simulink model "Feeder_1"  (Simulink 8.8)
settings: Solver=ode4  StartTime=0.0  StopTime=inf  FixedStep=Ts  RelTol=1e-3  EnableMultiTasking=on
PreLoadFcn:
  | Ts=125e-6;Core_Num = 0; np=1; nq=1; Vmin=.9;
PostLoadFcn:
  | Ts=125e-6;Core_Num = 0; np=1; nq=1; Vmin=.9;
InitFcn:
  | Ts=125e-6;Core_Num = 0; np=1; nq=1; Vmin=.9;
undefined symbols (not defined in the file or in its folder): another_event_name, DiscIntNeverNeededParam, I, j, Left, my_event_name, Right, type, V, X
libraries: powerlib x316, powerlib_meascontrol x227, simulink_extras x78, simulink x25, rtio_generic_c37_118 x22, ssn_lib x9, rtlab x6, powerlib_extras x3, artemis x1, rtio_opalrt_ml605ex1 x1, rtio_spectracom x1, rtio_generic_ethernet x1
(part 10 of 14)

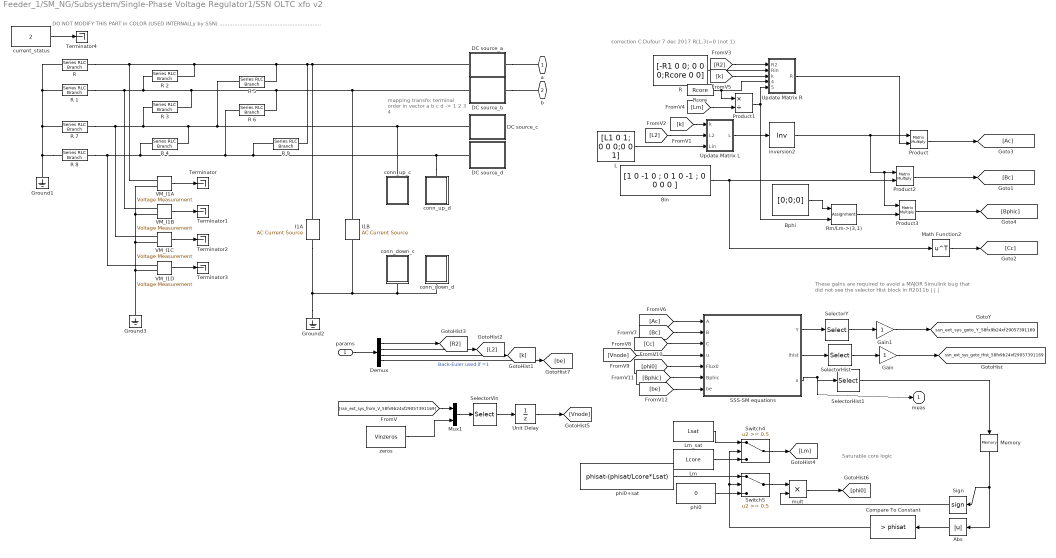
== system Feeder_1/SM_NG/Subsystem/Single-Phase Voltage Regulator1/SSN OLTC xfo v2 ==
  note: correction C.Dufour 7 dec 2017 R(1,3)=0 (not 1)
  note: These gains are required to avoid a MAJOR Simulink bug
      | that did not see the selector Hist block in R2011b
      | |
      | |
      | |
  note: Saturable core logic
  note: DO NOT MODIFY THIS PART in COLOR (USED INTERNALLy by SSN) .............................................................
  note: mapping transfo:
      | terminal    order in vector
      | a b c d -> 1 2 3 4
  params : Inport
  Abs : Abs
  Bin : Constant  Value="[1 0 -1  0 ; 0 1 0 -1 ; 0 0 0 0 ]"
  Bphi : Constant  Value=[0;0;0]  VectorParams1D=off
  Compare To Constant : simulink/Logic and Bit Operations/Compare To Constant  relop=>  const=phisat  OutDataTypeStr=uint8
  DC source_a : Subsystem  mask(SSN nodal point interface: DC-source){}
  DC source_b : Subsystem  mask(SSN nodal point interface: DC-source){}
  DC source_c : Subsystem  mask(SSN nodal point interface: DC-source){}
  DC source_d : Subsystem  mask(SSN nodal point interface: DC-source){}
  Demux : Demux
  Gain : Gain
  Gain1 : Gain
  Ground1 : powerlib/Elements/Ground  LConnTagsString=a
  Ground2 : powerlib/Elements/Ground  LConnTagsString=a
  Ground3 : powerlib/Elements/Ground  LConnTagsString=a
  I1A : powerlib/Electrical Sources/AC Current Source  Amplitude=0  Phase=0  Frequency=1928.3746  SampleTime=0  Measurements=None
  I1B : powerlib/Electrical Sources/AC Current Source  Amplitude=0  Phase=0  Frequency=1928.3746  SampleTime=0  Measurements=None
  L : Constant  Value=[L1 0 1; 0 0 0;0 0 1]
  Lm : Constant  Value=Lcore
  Lm_sat : Constant  Value=Lsat
  Math Function2 : Math  Operator=transpose  SaturateOnIntegerOverflow=on
  Memory : Memory
  Mux1 : Mux  Inputs=2
  Product : Product  Multiplication=Matrix(*)  RndMeth=Zero
  Product1 : Product  Inputs=*/  RndMeth=Zero
  Product2 : Product  Multiplication=Matrix(*)  RndMeth=Zero
  Product3 : Product  Multiplication=Matrix(*)  RndMeth=Zero
  R : Constant  Value=[-R1 0 0; 0 0 0;Rcore 0 0]
  R {,1..9} (10 alike) : powerlib/Elements/Series RLC Branch  LConnTagsString=__new0  RConnTagsString=__new0  BranchType=R  Resistance=1.23456789  Inductance=.5  SetiL0=off  InitialCurrent=0  Capacitance=1.0  Setx0=off  InitialVoltage=0  Measurements=None
  Rcore : Constant  Value=Rcore
  "Rm/Lm->(3,1) " : Assignment  NumberOfDimensions=2  IndexOptions=Index vector (dialog),Index vector (dialog)  Indices=3,1  OutputSizes=1,1
  SSS-SM equations : Subsystem
  SelectorHist : Selector  InputPortWidth=4  IndexOptions=Index vector (dialog)  Indices=hist_sel  OutputSizes=1
  SelectorHist1 : Selector  InputPortWidth=3  IndexOptions=Index vector (dialog)  Indices=3  OutputSizes=1
  SelectorVin : Selector  InputPortWidth=5  IndexOptions=Index vector (dialog)  Indices=vin_sel  OutputSizes=1
  SelectorY : Selector  NumberOfDimensions=2  InputPortWidth=4  IndexOptions=Index vector (dialog),Index vector (dialog)  Indices=hist_sel,hist_sel  OutputSizes=1,1
  Sign : Signum
  Switch4 : Switch  Threshold=0.5
  Switch5 : Switch  Threshold=0.5
  Terminator{,1..4} (5 alike) : Terminator
  Unit Delay : UnitDelay  SampleTime=Ts
  Update Matrix L : Subsystem
  Update Matrix R : Subsystem
  VM_I1A : powerlib/Measurements/Voltage Measurement  PhasorSimulation=off  OutputType=Complex  PSBequivalent=0
  VM_I1B : powerlib/Measurements/Voltage Measurement  PhasorSimulation=off  OutputType=Complex  PSBequivalent=0
  VM_I1C : powerlib/Measurements/Voltage Measurement  PhasorSimulation=off  OutputType=Complex  PSBequivalent=0
  VM_I1D : powerlib/Measurements/Voltage Measurement  PhasorSimulation=off  OutputType=Complex  PSBequivalent=0
  conn_down_c : Subsystem
  conn_down_d : Subsystem
  conn_up_c : Subsystem
  conn_up_d : Subsystem
  current_status : Constant  Value=2
  inversion2 : Product  Inputs=/  Multiplication=Matrix(*)  RndMeth=Zero
  mult : Product
  phi0 : Constant  Value=0
  phi0+sat : Constant  Value=phisat-(phisat/Lcore*Lsat)
  zeros : Constant  Value=Vinzeros
  a : PMIOPort  Port=1  Side=Left
  b : PMIOPort  Port=2  Side=Right
  meas : Outport  InitialOutput=0
  tag scope: ssn_ext_sys_goto_Hist_58fx9b24xf29057391169=global, ssn_ext_sys_goto_Y_58fx9b24xf29057391169=global
  wires:
  Gain1/1 -> [ssn_ext_sys_goto_Y_58fx9b24xf29057391169]
  Gain/1 -> [ssn_ext_sys_goto_Hist_58fx9b24xf29057391169]
  Sign/1 -> mult/2
  mult/1 -> [phi0]
  Switch5/1 -> mult/1
  Unit Delay/1 -> [Vnode]
  params/1 -> Demux/1
  Demux/1 -> [R2]
  Demux/2 -> [L2]
  Demux/3 -> [k]
  Abs/1 -> Compare To Constant/1
  Lm_sat/1 -> Switch4/1
  Lm/1 -> Switch4/3
  Memory/1 -> Abs/1, Sign/1
  phi0/1 -> Switch5/3
  phi0+sat/1 -> Switch5/1
  Switch4/1 -> [Lm]
  Compare To Constant/1 -> Switch4/2, Switch5/2
  [ssn_ext_sys_from_V_58fx9b24xf29057391169] -> Mux1/1
  zeros/1 -> Mux1/2
  SelectorVin/1 -> Unit Delay/1
  Mux1/1 -> SelectorVin/1
  current_status/1 -> Terminator4/1
  VM_I1D/1 -> Terminator3/1
  VM_I1C/1 -> Terminator2/1
  VM_I1B/1 -> Terminator1/1
  VM_I1A/1 -> Terminator/1
  L/1 -> Update Matrix L/3(Lin)
  [k] -> Update Matrix L/1(k)
  [L2] -> Update Matrix L/2(L2)
  Update Matrix L/1(L) -> inversion2/1
  R/1 -> Update Matrix R/2(Rin)
  [R2] -> Update Matrix R/1(R2)
  [k] -> Update Matrix R/3(k)
  Rcore/1 -> Update Matrix R/4(Rcore), Product1/1
  inversion2/1 -> Product2/1, Product3/1, Product/1
  [Lm] -> Product1/2
  Product1/1 -> Update Matrix R/5(Rcore/Lcore), "Rm/Lm->(3,1) "/2
  Bin/1 -> Math Function2/1, Product2/2
  Math Function2/1 -> [Cc]
  [Ac] -> SSS-SM equations/1(A)
  [Bc] -> SSS-SM equations/2(B)
  [Cc] -> SSS-SM equations/3(C)
  [Vnode] -> SSS-SM equations/4(u)
  [phi0] -> SSS-SM equations/5(Flux0)
  Bphi/1 -> "Rm/Lm->(3,1) "/1
  [Bphic] -> SSS-SM equations/6(Bphic)
  Product2/1 -> [Bc]
  "Rm/Lm->(3,1) "/1 -> Product3/2
  Update Matrix R/1(R) -> Product/2
  Product/1 -> [Ac]
  Product3/1 -> [Bphic]
  SSS-SM equations/3(x) -> SelectorHist1/1, meas/1
  SelectorHist1/1 -> Memory/1
  [be] -> SSS-SM equations/7(be)
  Demux/4 -> [be]  "Back-Euler used if =1"
  SSS-SM equations/2(Ihist) -> SelectorHist/1
  SSS-SM equations/1(Y) -> SelectorY/1
  SelectorY/1 -> Gain1/1
  SelectorHist/1 -> Gain/1
  connections:
  R 5/RConn1 -- VM_I1A/LConn1 -- "R "/RConn1 -- R 2/RConn1 -- I1A/RConn1 -- DC source_a/LConn1 -- R 9/RConn1
  R 3/RConn1 -- VM_I1B/LConn1 -- R 1/RConn1 -- R 2/LConn1 -- I1B/RConn1 -- DC source_b/LConn1 -- R 6/RConn1
  R 4/RConn1 -- VM_I1C/LConn1 -- R 7/RConn1 -- R 3/LConn1 -- conn_up_c/LConn1 -- DC source_c/LConn1 -- R 5/LConn1
  conn_up_d/LConn1 -- DC source_d/LConn1 -- R 9/LConn1 -- R 6/LConn1 -- VM_I1D/LConn1 -- R 8/RConn1 -- R 4/LConn1
  Ground3/LConn1 -- VM_I1C/LConn2 -- VM_I1A/LConn2 -- VM_I1B/LConn2 -- VM_I1D/LConn2
  DC source_b/RConn1 -- b/RConn1
  Ground2/LConn1 -- I1A/LConn1 -- I1B/LConn1 -- conn_down_c/RConn1 -- conn_down_d/RConn1
  DC source_a/RConn1 -- a/RConn1
  R 8/LConn1 -- Ground1/LConn1 -- R 7/LConn1 -- R 1/LConn1 -- "R "/LConn1

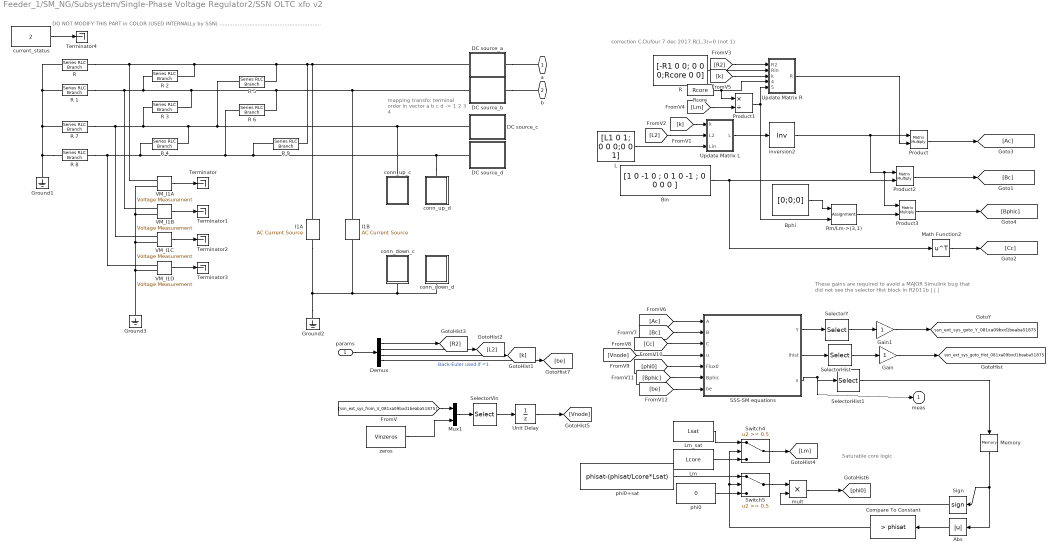
== system Feeder_1/SM_NG/Subsystem/Single-Phase Voltage Regulator2/SSN OLTC xfo v2 ==
  note: correction C.Dufour 7 dec 2017 R(1,3)=0 (not 1)
  note: These gains are required to avoid a MAJOR Simulink bug
      | that did not see the selector Hist block in R2011b
      | |
      | |
      | |
  note: Saturable core logic
  note: DO NOT MODIFY THIS PART in COLOR (USED INTERNALLy by SSN) .............................................................
  note: mapping transfo:
      | terminal    order in vector
      | a b c d -> 1 2 3 4
  params : Inport
  Abs : Abs
  Bin : Constant  Value="[1 0 -1  0 ; 0 1 0 -1 ; 0 0 0 0 ]"
  Bphi : Constant  Value=[0;0;0]  VectorParams1D=off
  Compare To Constant : simulink/Logic and Bit Operations/Compare To Constant  relop=>  const=phisat  OutDataTypeStr=uint8
  DC source_a : Subsystem  mask(SSN nodal point interface: DC-source){}
  DC source_b : Subsystem  mask(SSN nodal point interface: DC-source){}
  DC source_c : Subsystem  mask(SSN nodal point interface: DC-source){}
  DC source_d : Subsystem  mask(SSN nodal point interface: DC-source){}
  Demux : Demux
  Gain : Gain
  Gain1 : Gain
  Ground1 : powerlib/Elements/Ground  LConnTagsString=a
  Ground2 : powerlib/Elements/Ground  LConnTagsString=a
  Ground3 : powerlib/Elements/Ground  LConnTagsString=a
  I1A : powerlib/Electrical Sources/AC Current Source  Amplitude=0  Phase=0  Frequency=1928.3746  SampleTime=0  Measurements=None
  I1B : powerlib/Electrical Sources/AC Current Source  Amplitude=0  Phase=0  Frequency=1928.3746  SampleTime=0  Measurements=None
  L : Constant  Value=[L1 0 1; 0 0 0;0 0 1]
  Lm : Constant  Value=Lcore
  Lm_sat : Constant  Value=Lsat
  Math Function2 : Math  Operator=transpose  SaturateOnIntegerOverflow=on
  Memory : Memory
  Mux1 : Mux  Inputs=2
  Product : Product  Multiplication=Matrix(*)  RndMeth=Zero
  Product1 : Product  Inputs=*/  RndMeth=Zero
  Product2 : Product  Multiplication=Matrix(*)  RndMeth=Zero
  Product3 : Product  Multiplication=Matrix(*)  RndMeth=Zero
  R : Constant  Value=[-R1 0 0; 0 0 0;Rcore 0 0]
  R {,1..9} (10 alike) : powerlib/Elements/Series RLC Branch  LConnTagsString=__new0  RConnTagsString=__new0  BranchType=R  Resistance=1.23456789  Inductance=.5  SetiL0=off  InitialCurrent=0  Capacitance=1.0  Setx0=off  InitialVoltage=0  Measurements=None
  Rcore : Constant  Value=Rcore
  "Rm/Lm->(3,1) " : Assignment  NumberOfDimensions=2  IndexOptions=Index vector (dialog),Index vector (dialog)  Indices=3,1  OutputSizes=1,1
  SSS-SM equations : Subsystem
  SelectorHist : Selector  InputPortWidth=4  IndexOptions=Index vector (dialog)  Indices=hist_sel  OutputSizes=1
  SelectorHist1 : Selector  InputPortWidth=3  IndexOptions=Index vector (dialog)  Indices=3  OutputSizes=1
  SelectorVin : Selector  InputPortWidth=5  IndexOptions=Index vector (dialog)  Indices=vin_sel  OutputSizes=1
  SelectorY : Selector  NumberOfDimensions=2  InputPortWidth=4  IndexOptions=Index vector (dialog),Index vector (dialog)  Indices=hist_sel,hist_sel  OutputSizes=1,1
  Sign : Signum
  Switch4 : Switch  Threshold=0.5
  Switch5 : Switch  Threshold=0.5
  Terminator{,1..4} (5 alike) : Terminator
  Unit Delay : UnitDelay  SampleTime=Ts
  Update Matrix L : Subsystem
  Update Matrix R : Subsystem
  VM_I1A : powerlib/Measurements/Voltage Measurement  PhasorSimulation=off  OutputType=Complex  PSBequivalent=0
  VM_I1B : powerlib/Measurements/Voltage Measurement  PhasorSimulation=off  OutputType=Complex  PSBequivalent=0
  VM_I1C : powerlib/Measurements/Voltage Measurement  PhasorSimulation=off  OutputType=Complex  PSBequivalent=0
  VM_I1D : powerlib/Measurements/Voltage Measurement  PhasorSimulation=off  OutputType=Complex  PSBequivalent=0
  conn_down_c : Subsystem
  conn_down_d : Subsystem
  conn_up_c : Subsystem
  conn_up_d : Subsystem
  current_status : Constant  Value=2
  inversion2 : Product  Inputs=/  Multiplication=Matrix(*)  RndMeth=Zero
  mult : Product
  phi0 : Constant  Value=0
  phi0+sat : Constant  Value=phisat-(phisat/Lcore*Lsat)
  zeros : Constant  Value=Vinzeros
  a : PMIOPort  Port=1  Side=Left
  b : PMIOPort  Port=2  Side=Right
  meas : Outport  InitialOutput=0
  tag scope: ssn_ext_sys_goto_Hist_081xa09bxd1beaba51875=global, ssn_ext_sys_goto_Y_081xa09bxd1beaba51875=global
  wires:
  Gain1/1 -> [ssn_ext_sys_goto_Y_081xa09bxd1beaba51875]
  Gain/1 -> [ssn_ext_sys_goto_Hist_081xa09bxd1beaba51875]
  Sign/1 -> mult/2
  mult/1 -> [phi0]
  Switch5/1 -> mult/1
  Unit Delay/1 -> [Vnode]
  params/1 -> Demux/1
  Demux/1 -> [R2]
  Demux/2 -> [L2]
  Demux/3 -> [k]
  Abs/1 -> Compare To Constant/1
  Lm_sat/1 -> Switch4/1
  Lm/1 -> Switch4/3
  Memory/1 -> Abs/1, Sign/1
  phi0/1 -> Switch5/3
  phi0+sat/1 -> Switch5/1
  Switch4/1 -> [Lm]
  Compare To Constant/1 -> Switch4/2, Switch5/2
  [ssn_ext_sys_from_V_081xa09bxd1beaba51875] -> Mux1/1
  zeros/1 -> Mux1/2
  SelectorVin/1 -> Unit Delay/1
  Mux1/1 -> SelectorVin/1
  current_status/1 -> Terminator4/1
  VM_I1D/1 -> Terminator3/1
  VM_I1C/1 -> Terminator2/1
  VM_I1B/1 -> Terminator1/1
  VM_I1A/1 -> Terminator/1
  L/1 -> Update Matrix L/3(Lin)
  [k] -> Update Matrix L/1(k)
  [L2] -> Update Matrix L/2(L2)
  Update Matrix L/1(L) -> inversion2/1
  R/1 -> Update Matrix R/2(Rin)
  [R2] -> Update Matrix R/1(R2)
  [k] -> Update Matrix R/3(k)
  Rcore/1 -> Update Matrix R/4(Rcore), Product1/1
  inversion2/1 -> Product2/1, Product3/1, Product/1
  [Lm] -> Product1/2
  Product1/1 -> Update Matrix R/5(Rcore/Lcore), "Rm/Lm->(3,1) "/2
  Bin/1 -> Math Function2/1, Product2/2
  Math Function2/1 -> [Cc]
  [Ac] -> SSS-SM equations/1(A)
  [Bc] -> SSS-SM equations/2(B)
  [Cc] -> SSS-SM equations/3(C)
  [Vnode] -> SSS-SM equations/4(u)
  [phi0] -> SSS-SM equations/5(Flux0)
  Bphi/1 -> "Rm/Lm->(3,1) "/1
  [Bphic] -> SSS-SM equations/6(Bphic)
  Product2/1 -> [Bc]
  "Rm/Lm->(3,1) "/1 -> Product3/2
  Update Matrix R/1(R) -> Product/2
  Product/1 -> [Ac]
  Product3/1 -> [Bphic]
  SSS-SM equations/3(x) -> SelectorHist1/1, meas/1
  SelectorHist1/1 -> Memory/1
  [be] -> SSS-SM equations/7(be)
  Demux/4 -> [be]  "Back-Euler used if =1"
  SSS-SM equations/2(Ihist) -> SelectorHist/1
  SSS-SM equations/1(Y) -> SelectorY/1
  SelectorY/1 -> Gain1/1
  SelectorHist/1 -> Gain/1
  connections:
  R 5/RConn1 -- VM_I1A/LConn1 -- "R "/RConn1 -- R 2/RConn1 -- I1A/RConn1 -- DC source_a/LConn1 -- R 9/RConn1
  R 3/RConn1 -- VM_I1B/LConn1 -- R 1/RConn1 -- R 2/LConn1 -- I1B/RConn1 -- DC source_b/LConn1 -- R 6/RConn1
  R 4/RConn1 -- VM_I1C/LConn1 -- R 7/RConn1 -- R 3/LConn1 -- conn_up_c/LConn1 -- DC source_c/LConn1 -- R 5/LConn1
  conn_up_d/LConn1 -- DC source_d/LConn1 -- R 9/LConn1 -- R 6/LConn1 -- VM_I1D/LConn1 -- R 8/RConn1 -- R 4/LConn1
  Ground3/LConn1 -- VM_I1C/LConn2 -- VM_I1A/LConn2 -- VM_I1B/LConn2 -- VM_I1D/LConn2
  DC source_b/RConn1 -- b/RConn1
  Ground2/LConn1 -- I1A/LConn1 -- I1B/LConn1 -- conn_down_c/RConn1 -- conn_down_d/RConn1
  DC source_a/RConn1 -- a/RConn1
  R 8/LConn1 -- Ground1/LConn1 -- R 7/LConn1 -- R 1/LConn1 -- "R "/LConn1

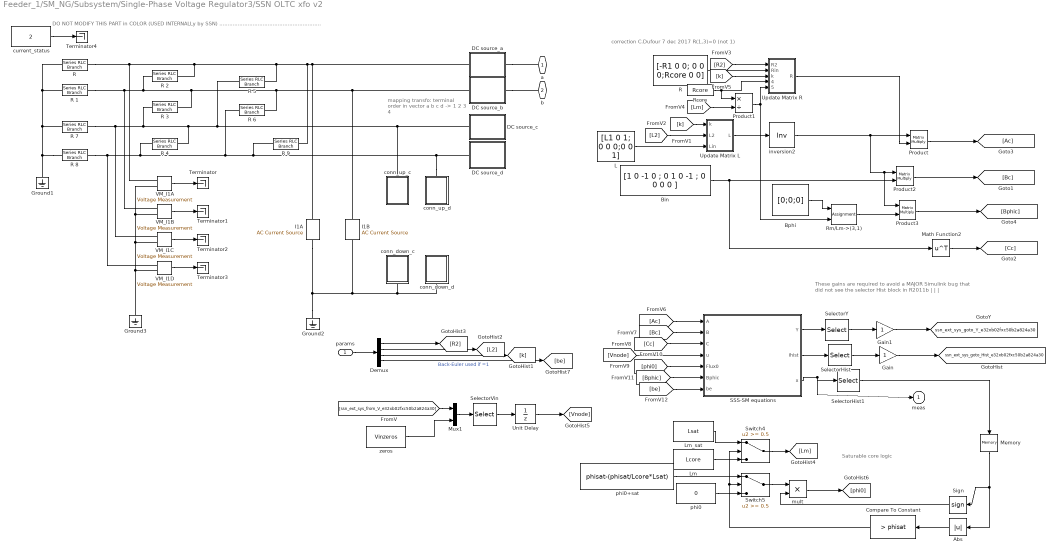
== system Feeder_1/SM_NG/Subsystem/Single-Phase Voltage Regulator3/SSN OLTC xfo v2 ==
  note: correction C.Dufour 7 dec 2017 R(1,3)=0 (not 1)
  note: These gains are required to avoid a MAJOR Simulink bug
      | that did not see the selector Hist block in R2011b
      | |
      | |
      | |
  note: Saturable core logic
  note: DO NOT MODIFY THIS PART in COLOR (USED INTERNALLy by SSN) .............................................................
  note: mapping transfo:
      | terminal    order in vector
      | a b c d -> 1 2 3 4
  params : Inport
  Abs : Abs
  Bin : Constant  Value="[1 0 -1  0 ; 0 1 0 -1 ; 0 0 0 0 ]"
  Bphi : Constant  Value=[0;0;0]  VectorParams1D=off
  Compare To Constant : simulink/Logic and Bit Operations/Compare To Constant  relop=>  const=phisat  OutDataTypeStr=uint8
  DC source_a : Subsystem  mask(SSN nodal point interface: DC-source){}
  DC source_b : Subsystem  mask(SSN nodal point interface: DC-source){}
  DC source_c : Subsystem  mask(SSN nodal point interface: DC-source){}
  DC source_d : Subsystem  mask(SSN nodal point interface: DC-source){}
  Demux : Demux
  Gain : Gain
  Gain1 : Gain
  Ground1 : powerlib/Elements/Ground  LConnTagsString=a
  Ground2 : powerlib/Elements/Ground  LConnTagsString=a
  Ground3 : powerlib/Elements/Ground  LConnTagsString=a
  I1A : powerlib/Electrical Sources/AC Current Source  Amplitude=0  Phase=0  Frequency=1928.3746  SampleTime=0  Measurements=None
  I1B : powerlib/Electrical Sources/AC Current Source  Amplitude=0  Phase=0  Frequency=1928.3746  SampleTime=0  Measurements=None
  L : Constant  Value=[L1 0 1; 0 0 0;0 0 1]
  Lm : Constant  Value=Lcore
  Lm_sat : Constant  Value=Lsat
  Math Function2 : Math  Operator=transpose  SaturateOnIntegerOverflow=on
  Memory : Memory
  Mux1 : Mux  Inputs=2
  Product : Product  Multiplication=Matrix(*)  RndMeth=Zero
  Product1 : Product  Inputs=*/  RndMeth=Zero
  Product2 : Product  Multiplication=Matrix(*)  RndMeth=Zero
  Product3 : Product  Multiplication=Matrix(*)  RndMeth=Zero
  R : Constant  Value=[-R1 0 0; 0 0 0;Rcore 0 0]
  R {,1..9} (10 alike) : powerlib/Elements/Series RLC Branch  LConnTagsString=__new0  RConnTagsString=__new0  BranchType=R  Resistance=1.23456789  Inductance=.5  SetiL0=off  InitialCurrent=0  Capacitance=1.0  Setx0=off  InitialVoltage=0  Measurements=None
  Rcore : Constant  Value=Rcore
  "Rm/Lm->(3,1) " : Assignment  NumberOfDimensions=2  IndexOptions=Index vector (dialog),Index vector (dialog)  Indices=3,1  OutputSizes=1,1
  SSS-SM equations : Subsystem
  SelectorHist : Selector  InputPortWidth=4  IndexOptions=Index vector (dialog)  Indices=hist_sel  OutputSizes=1
  SelectorHist1 : Selector  InputPortWidth=3  IndexOptions=Index vector (dialog)  Indices=3  OutputSizes=1
  SelectorVin : Selector  InputPortWidth=5  IndexOptions=Index vector (dialog)  Indices=vin_sel  OutputSizes=1
  SelectorY : Selector  NumberOfDimensions=2  InputPortWidth=4  IndexOptions=Index vector (dialog),Index vector (dialog)  Indices=hist_sel,hist_sel  OutputSizes=1,1
  Sign : Signum
  Switch4 : Switch  Threshold=0.5
  Switch5 : Switch  Threshold=0.5
  Terminator{,1..4} (5 alike) : Terminator
  Unit Delay : UnitDelay  SampleTime=Ts
  Update Matrix L : Subsystem
  Update Matrix R : Subsystem
  VM_I1A : powerlib/Measurements/Voltage Measurement  PhasorSimulation=off  OutputType=Complex  PSBequivalent=0
  VM_I1B : powerlib/Measurements/Voltage Measurement  PhasorSimulation=off  OutputType=Complex  PSBequivalent=0
  VM_I1C : powerlib/Measurements/Voltage Measurement  PhasorSimulation=off  OutputType=Complex  PSBequivalent=0
  VM_I1D : powerlib/Measurements/Voltage Measurement  PhasorSimulation=off  OutputType=Complex  PSBequivalent=0
  conn_down_c : Subsystem
  conn_down_d : Subsystem
  conn_up_c : Subsystem
  conn_up_d : Subsystem
  current_status : Constant  Value=2
  inversion2 : Product  Inputs=/  Multiplication=Matrix(*)  RndMeth=Zero
  mult : Product
  phi0 : Constant  Value=0
  phi0+sat : Constant  Value=phisat-(phisat/Lcore*Lsat)
  zeros : Constant  Value=Vinzeros
  a : PMIOPort  Port=1  Side=Left
  b : PMIOPort  Port=2  Side=Right
  meas : Outport  InitialOutput=0
  tag scope: ssn_ext_sys_goto_Hist_e32xb02fxc50b2a824a30=global, ssn_ext_sys_goto_Y_e32xb02fxc50b2a824a30=global
  wires:
  Gain1/1 -> [ssn_ext_sys_goto_Y_e32xb02fxc50b2a824a30]
  Gain/1 -> [ssn_ext_sys_goto_Hist_e32xb02fxc50b2a824a30]
  Sign/1 -> mult/2
  mult/1 -> [phi0]
  Switch5/1 -> mult/1
  Unit Delay/1 -> [Vnode]
  params/1 -> Demux/1
  Demux/1 -> [R2]
  Demux/2 -> [L2]
  Demux/3 -> [k]
  Abs/1 -> Compare To Constant/1
  Lm_sat/1 -> Switch4/1
  Lm/1 -> Switch4/3
  Memory/1 -> Abs/1, Sign/1
  phi0/1 -> Switch5/3
  phi0+sat/1 -> Switch5/1
  Switch4/1 -> [Lm]
  Compare To Constant/1 -> Switch4/2, Switch5/2
  [ssn_ext_sys_from_V_e32xb02fxc50b2a824a30] -> Mux1/1
  zeros/1 -> Mux1/2
  SelectorVin/1 -> Unit Delay/1
  Mux1/1 -> SelectorVin/1
  current_status/1 -> Terminator4/1
  VM_I1D/1 -> Terminator3/1
  VM_I1C/1 -> Terminator2/1
  VM_I1B/1 -> Terminator1/1
  VM_I1A/1 -> Terminator/1
  L/1 -> Update Matrix L/3(Lin)
  [k] -> Update Matrix L/1(k)
  [L2] -> Update Matrix L/2(L2)
  Update Matrix L/1(L) -> inversion2/1
  R/1 -> Update Matrix R/2(Rin)
  [R2] -> Update Matrix R/1(R2)
  [k] -> Update Matrix R/3(k)
  Rcore/1 -> Update Matrix R/4(Rcore), Product1/1
  inversion2/1 -> Product2/1, Product3/1, Product/1
  [Lm] -> Product1/2
  Product1/1 -> Update Matrix R/5(Rcore/Lcore), "Rm/Lm->(3,1) "/2
  Bin/1 -> Math Function2/1, Product2/2
  Math Function2/1 -> [Cc]
  [Ac] -> SSS-SM equations/1(A)
  [Bc] -> SSS-SM equations/2(B)
  [Cc] -> SSS-SM equations/3(C)
  [Vnode] -> SSS-SM equations/4(u)
  [phi0] -> SSS-SM equations/5(Flux0)
  Bphi/1 -> "Rm/Lm->(3,1) "/1
  [Bphic] -> SSS-SM equations/6(Bphic)
  Product2/1 -> [Bc]
  "Rm/Lm->(3,1) "/1 -> Product3/2
  Update Matrix R/1(R) -> Product/2
  Product/1 -> [Ac]
  Product3/1 -> [Bphic]
  SSS-SM equations/3(x) -> SelectorHist1/1, meas/1
  SelectorHist1/1 -> Memory/1
  [be] -> SSS-SM equations/7(be)
  Demux/4 -> [be]  "Back-Euler used if =1"
  SSS-SM equations/2(Ihist) -> SelectorHist/1
  SSS-SM equations/1(Y) -> SelectorY/1
  SelectorY/1 -> Gain1/1
  SelectorHist/1 -> Gain/1
  connections:
  R 5/RConn1 -- VM_I1A/LConn1 -- "R "/RConn1 -- R 2/RConn1 -- I1A/RConn1 -- DC source_a/LConn1 -- R 9/RConn1
  R 3/RConn1 -- VM_I1B/LConn1 -- R 1/RConn1 -- R 2/LConn1 -- I1B/RConn1 -- DC source_b/LConn1 -- R 6/RConn1
  R 4/RConn1 -- VM_I1C/LConn1 -- R 7/RConn1 -- R 3/LConn1 -- conn_up_c/LConn1 -- DC source_c/LConn1 -- R 5/LConn1
  conn_up_d/LConn1 -- DC source_d/LConn1 -- R 9/LConn1 -- R 6/LConn1 -- VM_I1D/LConn1 -- R 8/RConn1 -- R 4/LConn1
  Ground3/LConn1 -- VM_I1C/LConn2 -- VM_I1A/LConn2 -- VM_I1B/LConn2 -- VM_I1D/LConn2
  DC source_b/RConn1 -- b/RConn1
  Ground2/LConn1 -- I1A/LConn1 -- I1B/LConn1 -- conn_down_c/RConn1 -- conn_down_d/RConn1
  DC source_a/RConn1 -- a/RConn1
  R 8/LConn1 -- Ground1/LConn1 -- R 7/LConn1 -- R 1/LConn1 -- "R "/LConn1

== system Feeder_1/SS_PMU/Subsystem1/Subsystem/Subsystem1 ==
  Measurements : Inport
  Degree to radian1 : Subsystem
  Mux1 : Mux
  Selector5 : Selector  InputPortWidth=12  IndexOptions=Index vector (dialog)  Indices=[1 3 5]  OutputSizes=1
  Selector6 : Selector  InputPortWidth=12  IndexOptions=Index vector (dialog)  Indices=[7 9 11]  OutputSizes=1
  Selector7 : Selector  InputPortWidth=6  IndexOptions=Index vector (dialog)  Indices=[1 2 3]  OutputSizes=1
  Selector8 : Selector  InputPortWidth=6  IndexOptions=Index vector (dialog)  Indices=[4 5 6]  OutputSizes=1
  Selector9 : Selector  InputPortWidth=12  IndexOptions=Index vector (dialog)  Indices=[2 4 6 8 10 12]  OutputSizes=1
  Subsystem : Subsystem
  Phasors_abc : Outport
  Phasors_Freq : Outport  Port=2
  Phasors_DTFreq : Outport  Port=3
  wires:
  Subsystem/2(Phasors_freq) -> Phasors_Freq/1
  Subsystem/3(Phasors_dtfreq1) -> Phasors_DTFreq/1
  Selector5/1 -> Mux1/1
  Mux1/1 -> Phasors_abc/1
  Selector7/1 -> Mux1/2
  Subsystem/1(Phasors_60Hz) -> Selector5/1, Selector6/1, Selector9/1
  Selector8/1 -> Mux1/4
  Selector6/1 -> Mux1/3
  Measurements/1 -> Subsystem/1(Measurements1)
  Selector9/1 -> Degree to radian1/1(Degree)
  Degree to radian1/1(Radian) -> Selector7/1, Selector8/1

== system Feeder_1/SS_PMU/Subsystem10/Subsystem/Subsystem1 ==
  Measurements : Inport
  Degree to radian1 : Subsystem
  Mux1 : Mux
  Selector5 : Selector  InputPortWidth=12  IndexOptions=Index vector (dialog)  Indices=[1 3 5]  OutputSizes=1
  Selector6 : Selector  InputPortWidth=12  IndexOptions=Index vector (dialog)  Indices=[7 9 11]  OutputSizes=1
  Selector7 : Selector  InputPortWidth=6  IndexOptions=Index vector (dialog)  Indices=[1 2 3]  OutputSizes=1
  Selector8 : Selector  InputPortWidth=6  IndexOptions=Index vector (dialog)  Indices=[4 5 6]  OutputSizes=1
  Selector9 : Selector  InputPortWidth=12  IndexOptions=Index vector (dialog)  Indices=[2 4 6 8 10 12]  OutputSizes=1
  Subsystem : Subsystem
  Phasors_abc : Outport
  Phasors_Freq : Outport  Port=2
  Phasors_DTFreq : Outport  Port=3
  wires:
  Subsystem/2(Phasors_freq) -> Phasors_Freq/1
  Subsystem/3(Phasors_dtfreq1) -> Phasors_DTFreq/1
  Selector5/1 -> Mux1/1
  Mux1/1 -> Phasors_abc/1
  Selector7/1 -> Mux1/2
  Subsystem/1(Phasors_60Hz) -> Selector5/1, Selector6/1, Selector9/1
  Selector8/1 -> Mux1/4
  Selector6/1 -> Mux1/3
  Measurements/1 -> Subsystem/1(Measurements1)
  Selector9/1 -> Degree to radian1/1(Degree)
  Degree to radian1/1(Radian) -> Selector7/1, Selector8/1

== system Feeder_1/SS_PMU/Subsystem11/Subsystem/Subsystem1 ==
  Measurements : Inport
  Degree to radian1 : Subsystem
  Mux1 : Mux
  Selector5 : Selector  InputPortWidth=12  IndexOptions=Index vector (dialog)  Indices=[1 3 5]  OutputSizes=1
  Selector6 : Selector  InputPortWidth=12  IndexOptions=Index vector (dialog)  Indices=[7 9 11]  OutputSizes=1
  Selector7 : Selector  InputPortWidth=6  IndexOptions=Index vector (dialog)  Indices=[1 2 3]  OutputSizes=1
  Selector8 : Selector  InputPortWidth=6  IndexOptions=Index vector (dialog)  Indices=[4 5 6]  OutputSizes=1
  Selector9 : Selector  InputPortWidth=12  IndexOptions=Index vector (dialog)  Indices=[2 4 6 8 10 12]  OutputSizes=1
  Subsystem : Subsystem
  Phasors_abc : Outport
  Phasors_Freq : Outport  Port=2
  Phasors_DTFreq : Outport  Port=3
  wires:
  Subsystem/2(Phasors_freq) -> Phasors_Freq/1
  Subsystem/3(Phasors_dtfreq1) -> Phasors_DTFreq/1
  Selector5/1 -> Mux1/1
  Mux1/1 -> Phasors_abc/1
  Selector7/1 -> Mux1/2
  Subsystem/1(Phasors_60Hz) -> Selector5/1, Selector6/1, Selector9/1
  Selector8/1 -> Mux1/4
  Selector6/1 -> Mux1/3
  Measurements/1 -> Subsystem/1(Measurements1)
  Selector9/1 -> Degree to radian1/1(Degree)
  Degree to radian1/1(Radian) -> Selector7/1, Selector8/1

== system Feeder_1/SS_PMU/Subsystem12/Subsystem/Subsystem1 ==
  Measurements : Inport
  Degree to radian1 : Subsystem
  Mux1 : Mux
  Selector5 : Selector  InputPortWidth=12  IndexOptions=Index vector (dialog)  Indices=[1 3 5]  OutputSizes=1
  Selector6 : Selector  InputPortWidth=12  IndexOptions=Index vector (dialog)  Indices=[7 9 11]  OutputSizes=1
  Selector7 : Selector  InputPortWidth=6  IndexOptions=Index vector (dialog)  Indices=[1 2 3]  OutputSizes=1
  Selector8 : Selector  InputPortWidth=6  IndexOptions=Index vector (dialog)  Indices=[4 5 6]  OutputSizes=1
  Selector9 : Selector  InputPortWidth=12  IndexOptions=Index vector (dialog)  Indices=[2 4 6 8 10 12]  OutputSizes=1
  Subsystem : Subsystem
  Phasors_abc : Outport
  Phasors_Freq : Outport  Port=2
  Phasors_DTFreq : Outport  Port=3
  wires:
  Subsystem/2(Phasors_freq) -> Phasors_Freq/1
  Subsystem/3(Phasors_dtfreq1) -> Phasors_DTFreq/1
  Selector5/1 -> Mux1/1
  Mux1/1 -> Phasors_abc/1
  Selector7/1 -> Mux1/2
  Subsystem/1(Phasors_60Hz) -> Selector5/1, Selector6/1, Selector9/1
  Selector8/1 -> Mux1/4
  Selector6/1 -> Mux1/3
  Measurements/1 -> Subsystem/1(Measurements1)
  Selector9/1 -> Degree to radian1/1(Degree)
  Degree to radian1/1(Radian) -> Selector7/1, Selector8/1

== system Feeder_1/SS_PMU/Subsystem13/Subsystem/Subsystem1 ==
  Measurements : Inport
  Degree to radian1 : Subsystem
  Mux1 : Mux
  Selector5 : Selector  InputPortWidth=12  IndexOptions=Index vector (dialog)  Indices=[1 3 5]  OutputSizes=1
  Selector6 : Selector  InputPortWidth=12  IndexOptions=Index vector (dialog)  Indices=[7 9 11]  OutputSizes=1
  Selector7 : Selector  InputPortWidth=6  IndexOptions=Index vector (dialog)  Indices=[1 2 3]  OutputSizes=1
  Selector8 : Selector  InputPortWidth=6  IndexOptions=Index vector (dialog)  Indices=[4 5 6]  OutputSizes=1
  Selector9 : Selector  InputPortWidth=12  IndexOptions=Index vector (dialog)  Indices=[2 4 6 8 10 12]  OutputSizes=1
  Subsystem : Subsystem
  Phasors_abc : Outport
  Phasors_Freq : Outport  Port=2
  Phasors_DTFreq : Outport  Port=3
  wires:
  Subsystem/2(Phasors_freq) -> Phasors_Freq/1
  Subsystem/3(Phasors_dtfreq1) -> Phasors_DTFreq/1
  Selector5/1 -> Mux1/1
  Mux1/1 -> Phasors_abc/1
  Selector7/1 -> Mux1/2
  Subsystem/1(Phasors_60Hz) -> Selector5/1, Selector6/1, Selector9/1
  Selector8/1 -> Mux1/4
  Selector6/1 -> Mux1/3
  Measurements/1 -> Subsystem/1(Measurements1)
  Selector9/1 -> Degree to radian1/1(Degree)
  Degree to radian1/1(Radian) -> Selector7/1, Selector8/1

== system Feeder_1/SS_PMU/Subsystem14/Subsystem/Subsystem1 ==
  Measurements : Inport
  Degree to radian1 : Subsystem
  Mux1 : Mux
  Selector5 : Selector  InputPortWidth=12  IndexOptions=Index vector (dialog)  Indices=[1 3 5]  OutputSizes=1
  Selector6 : Selector  InputPortWidth=12  IndexOptions=Index vector (dialog)  Indices=[7 9 11]  OutputSizes=1
  Selector7 : Selector  InputPortWidth=6  IndexOptions=Index vector (dialog)  Indices=[1 2 3]  OutputSizes=1
  Selector8 : Selector  InputPortWidth=6  IndexOptions=Index vector (dialog)  Indices=[4 5 6]  OutputSizes=1
  Selector9 : Selector  InputPortWidth=12  IndexOptions=Index vector (dialog)  Indices=[2 4 6 8 10 12]  OutputSizes=1
  Subsystem : Subsystem
  Phasors_abc : Outport
  Phasors_Freq : Outport  Port=2
  Phasors_DTFreq : Outport  Port=3
  wires:
  Subsystem/2(Phasors_freq) -> Phasors_Freq/1
  Subsystem/3(Phasors_dtfreq1) -> Phasors_DTFreq/1
  Selector5/1 -> Mux1/1
  Mux1/1 -> Phasors_abc/1
  Selector7/1 -> Mux1/2
  Subsystem/1(Phasors_60Hz) -> Selector5/1, Selector6/1, Selector9/1
  Selector8/1 -> Mux1/4
  Selector6/1 -> Mux1/3
  Measurements/1 -> Subsystem/1(Measurements1)
  Selector9/1 -> Degree to radian1/1(Degree)
  Degree to radian1/1(Radian) -> Selector7/1, Selector8/1

== system Feeder_1/SS_PMU/Subsystem15/Subsystem/Subsystem1 ==
  Measurements : Inport
  Degree to radian1 : Subsystem
  Mux1 : Mux
  Selector5 : Selector  InputPortWidth=12  IndexOptions=Index vector (dialog)  Indices=[1 3 5]  OutputSizes=1
  Selector6 : Selector  InputPortWidth=12  IndexOptions=Index vector (dialog)  Indices=[7 9 11]  OutputSizes=1
  Selector7 : Selector  InputPortWidth=6  IndexOptions=Index vector (dialog)  Indices=[1 2 3]  OutputSizes=1
  Selector8 : Selector  InputPortWidth=6  IndexOptions=Index vector (dialog)  Indices=[4 5 6]  OutputSizes=1
  Selector9 : Selector  InputPortWidth=12  IndexOptions=Index vector (dialog)  Indices=[2 4 6 8 10 12]  OutputSizes=1
  Subsystem : Subsystem
  Phasors_abc : Outport
  Phasors_Freq : Outport  Port=2
  Phasors_DTFreq : Outport  Port=3
  wires:
  Subsystem/2(Phasors_freq) -> Phasors_Freq/1
  Subsystem/3(Phasors_dtfreq1) -> Phasors_DTFreq/1
  Selector5/1 -> Mux1/1
  Mux1/1 -> Phasors_abc/1
  Selector7/1 -> Mux1/2
  Subsystem/1(Phasors_60Hz) -> Selector5/1, Selector6/1, Selector9/1
  Selector8/1 -> Mux1/4
  Selector6/1 -> Mux1/3
  Measurements/1 -> Subsystem/1(Measurements1)
  Selector9/1 -> Degree to radian1/1(Degree)
  Degree to radian1/1(Radian) -> Selector7/1, Selector8/1

== system Feeder_1/SS_PMU/Subsystem16/Subsystem/Subsystem1 ==
  Measurements : Inport
  Degree to radian1 : Subsystem
  Mux1 : Mux
  Selector5 : Selector  InputPortWidth=12  IndexOptions=Index vector (dialog)  Indices=[1 3 5]  OutputSizes=1
  Selector6 : Selector  InputPortWidth=12  IndexOptions=Index vector (dialog)  Indices=[7 9 11]  OutputSizes=1
  Selector7 : Selector  InputPortWidth=6  IndexOptions=Index vector (dialog)  Indices=[1 2 3]  OutputSizes=1
  Selector8 : Selector  InputPortWidth=6  IndexOptions=Index vector (dialog)  Indices=[4 5 6]  OutputSizes=1
  Selector9 : Selector  InputPortWidth=12  IndexOptions=Index vector (dialog)  Indices=[2 4 6 8 10 12]  OutputSizes=1
  Subsystem : Subsystem
  Phasors_abc : Outport
  Phasors_Freq : Outport  Port=2
  Phasors_DTFreq : Outport  Port=3
  wires:
  Subsystem/2(Phasors_freq) -> Phasors_Freq/1
  Subsystem/3(Phasors_dtfreq1) -> Phasors_DTFreq/1
  Selector5/1 -> Mux1/1
  Mux1/1 -> Phasors_abc/1
  Selector7/1 -> Mux1/2
  Subsystem/1(Phasors_60Hz) -> Selector5/1, Selector6/1, Selector9/1
  Selector8/1 -> Mux1/4
  Selector6/1 -> Mux1/3
  Measurements/1 -> Subsystem/1(Measurements1)
  Selector9/1 -> Degree to radian1/1(Degree)
  Degree to radian1/1(Radian) -> Selector7/1, Selector8/1

== system Feeder_1/SS_PMU/Subsystem17/Subsystem/Subsystem1 ==
  Measurements : Inport
  Degree to radian1 : Subsystem
  Mux1 : Mux
  Selector5 : Selector  InputPortWidth=12  IndexOptions=Index vector (dialog)  Indices=[1 3 5]  OutputSizes=1
  Selector6 : Selector  InputPortWidth=12  IndexOptions=Index vector (dialog)  Indices=[7 9 11]  OutputSizes=1
  Selector7 : Selector  InputPortWidth=6  IndexOptions=Index vector (dialog)  Indices=[1 2 3]  OutputSizes=1
  Selector8 : Selector  InputPortWidth=6  IndexOptions=Index vector (dialog)  Indices=[4 5 6]  OutputSizes=1
  Selector9 : Selector  InputPortWidth=12  IndexOptions=Index vector (dialog)  Indices=[2 4 6 8 10 12]  OutputSizes=1
  Subsystem : Subsystem
  Phasors_abc : Outport
  Phasors_Freq : Outport  Port=2
  Phasors_DTFreq : Outport  Port=3
  wires:
  Subsystem/2(Phasors_freq) -> Phasors_Freq/1
  Subsystem/3(Phasors_dtfreq1) -> Phasors_DTFreq/1
  Selector5/1 -> Mux1/1
  Mux1/1 -> Phasors_abc/1
  Selector7/1 -> Mux1/2
  Subsystem/1(Phasors_60Hz) -> Selector5/1, Selector6/1, Selector9/1
  Selector8/1 -> Mux1/4
  Selector6/1 -> Mux1/3
  Measurements/1 -> Subsystem/1(Measurements1)
  Selector9/1 -> Degree to radian1/1(Degree)
  Degree to radian1/1(Radian) -> Selector7/1, Selector8/1

== system Feeder_1/SS_PMU/Subsystem18/Subsystem/Subsystem1 ==
  Measurements : Inport
  Degree to radian1 : Subsystem
  Mux1 : Mux
  Selector5 : Selector  InputPortWidth=12  IndexOptions=Index vector (dialog)  Indices=[1 3 5]  OutputSizes=1
  Selector6 : Selector  InputPortWidth=12  IndexOptions=Index vector (dialog)  Indices=[7 9 11]  OutputSizes=1
  Selector7 : Selector  InputPortWidth=6  IndexOptions=Index vector (dialog)  Indices=[1 2 3]  OutputSizes=1
  Selector8 : Selector  InputPortWidth=6  IndexOptions=Index vector (dialog)  Indices=[4 5 6]  OutputSizes=1
  Selector9 : Selector  InputPortWidth=12  IndexOptions=Index vector (dialog)  Indices=[2 4 6 8 10 12]  OutputSizes=1
  Subsystem : Subsystem
  Phasors_abc : Outport
  Phasors_Freq : Outport  Port=2
  Phasors_DTFreq : Outport  Port=3
  wires:
  Subsystem/2(Phasors_freq) -> Phasors_Freq/1
  Subsystem/3(Phasors_dtfreq1) -> Phasors_DTFreq/1
  Selector5/1 -> Mux1/1
  Mux1/1 -> Phasors_abc/1
  Selector7/1 -> Mux1/2
  Subsystem/1(Phasors_60Hz) -> Selector5/1, Selector6/1, Selector9/1
  Selector8/1 -> Mux1/4
  Selector6/1 -> Mux1/3
  Measurements/1 -> Subsystem/1(Measurements1)
  Selector9/1 -> Degree to radian1/1(Degree)
  Degree to radian1/1(Radian) -> Selector7/1, Selector8/1

== system Feeder_1/SS_PMU/Subsystem19/Subsystem/Subsystem1 ==
  Measurements : Inport
  Degree to radian1 : Subsystem
  Mux1 : Mux
  Selector5 : Selector  InputPortWidth=12  IndexOptions=Index vector (dialog)  Indices=[1 3 5]  OutputSizes=1
  Selector6 : Selector  InputPortWidth=12  IndexOptions=Index vector (dialog)  Indices=[7 9 11]  OutputSizes=1
  Selector7 : Selector  InputPortWidth=6  IndexOptions=Index vector (dialog)  Indices=[1 2 3]  OutputSizes=1
  Selector8 : Selector  InputPortWidth=6  IndexOptions=Index vector (dialog)  Indices=[4 5 6]  OutputSizes=1
  Selector9 : Selector  InputPortWidth=12  IndexOptions=Index vector (dialog)  Indices=[2 4 6 8 10 12]  OutputSizes=1
  Subsystem : Subsystem
  Phasors_abc : Outport
  Phasors_Freq : Outport  Port=2
  Phasors_DTFreq : Outport  Port=3
  wires:
  Subsystem/2(Phasors_freq) -> Phasors_Freq/1
  Subsystem/3(Phasors_dtfreq1) -> Phasors_DTFreq/1
  Selector5/1 -> Mux1/1
  Mux1/1 -> Phasors_abc/1
  Selector7/1 -> Mux1/2
  Subsystem/1(Phasors_60Hz) -> Selector5/1, Selector6/1, Selector9/1
  Selector8/1 -> Mux1/4
  Selector6/1 -> Mux1/3
  Measurements/1 -> Subsystem/1(Measurements1)
  Selector9/1 -> Degree to radian1/1(Degree)
  Degree to radian1/1(Radian) -> Selector7/1, Selector8/1

== system Feeder_1/SS_PMU/Subsystem2/Subsystem/Subsystem1 ==
  Measurements : Inport
  Degree to radian1 : Subsystem
  Mux1 : Mux
  Selector5 : Selector  InputPortWidth=12  IndexOptions=Index vector (dialog)  Indices=[1 3 5]  OutputSizes=1
  Selector6 : Selector  InputPortWidth=12  IndexOptions=Index vector (dialog)  Indices=[7 9 11]  OutputSizes=1
  Selector7 : Selector  InputPortWidth=6  IndexOptions=Index vector (dialog)  Indices=[1 2 3]  OutputSizes=1
  Selector8 : Selector  InputPortWidth=6  IndexOptions=Index vector (dialog)  Indices=[4 5 6]  OutputSizes=1
  Selector9 : Selector  InputPortWidth=12  IndexOptions=Index vector (dialog)  Indices=[2 4 6 8 10 12]  OutputSizes=1
  Subsystem : Subsystem
  Phasors_abc : Outport
  Phasors_Freq : Outport  Port=2
  Phasors_DTFreq : Outport  Port=3
  wires:
  Subsystem/2(Phasors_freq) -> Phasors_Freq/1
  Subsystem/3(Phasors_dtfreq1) -> Phasors_DTFreq/1
  Selector5/1 -> Mux1/1
  Mux1/1 -> Phasors_abc/1
  Selector7/1 -> Mux1/2
  Subsystem/1(Phasors_60Hz) -> Selector5/1, Selector6/1, Selector9/1
  Selector8/1 -> Mux1/4
  Selector6/1 -> Mux1/3
  Measurements/1 -> Subsystem/1(Measurements1)
  Selector9/1 -> Degree to radian1/1(Degree)
  Degree to radian1/1(Radian) -> Selector7/1, Selector8/1

== system Feeder_1/SS_PMU/Subsystem20/Subsystem/Subsystem1 ==
  Measurements : Inport
  Degree to radian1 : Subsystem
  Mux1 : Mux
  Selector5 : Selector  InputPortWidth=12  IndexOptions=Index vector (dialog)  Indices=[1 3 5]  OutputSizes=1
  Selector6 : Selector  InputPortWidth=12  IndexOptions=Index vector (dialog)  Indices=[7 9 11]  OutputSizes=1
  Selector7 : Selector  InputPortWidth=6  IndexOptions=Index vector (dialog)  Indices=[1 2 3]  OutputSizes=1
  Selector8 : Selector  InputPortWidth=6  IndexOptions=Index vector (dialog)  Indices=[4 5 6]  OutputSizes=1
  Selector9 : Selector  InputPortWidth=12  IndexOptions=Index vector (dialog)  Indices=[2 4 6 8 10 12]  OutputSizes=1
  Subsystem : Subsystem
  Phasors_abc : Outport
  Phasors_Freq : Outport  Port=2
  Phasors_DTFreq : Outport  Port=3
  wires:
  Subsystem/2(Phasors_freq) -> Phasors_Freq/1
  Subsystem/3(Phasors_dtfreq1) -> Phasors_DTFreq/1
  Selector5/1 -> Mux1/1
  Mux1/1 -> Phasors_abc/1
  Selector7/1 -> Mux1/2
  Subsystem/1(Phasors_60Hz) -> Selector5/1, Selector6/1, Selector9/1
  Selector8/1 -> Mux1/4
  Selector6/1 -> Mux1/3
  Measurements/1 -> Subsystem/1(Measurements1)
  Selector9/1 -> Degree to radian1/1(Degree)
  Degree to radian1/1(Radian) -> Selector7/1, Selector8/1

== system Feeder_1/SS_PMU/Subsystem21/Subsystem/Subsystem1 ==
  Measurements : Inport
  Degree to radian1 : Subsystem
  Mux1 : Mux
  Selector5 : Selector  InputPortWidth=12  IndexOptions=Index vector (dialog)  Indices=[1 3 5]  OutputSizes=1
  Selector6 : Selector  InputPortWidth=12  IndexOptions=Index vector (dialog)  Indices=[7 9 11]  OutputSizes=1
  Selector7 : Selector  InputPortWidth=6  IndexOptions=Index vector (dialog)  Indices=[1 2 3]  OutputSizes=1
  Selector8 : Selector  InputPortWidth=6  IndexOptions=Index vector (dialog)  Indices=[4 5 6]  OutputSizes=1
  Selector9 : Selector  InputPortWidth=12  IndexOptions=Index vector (dialog)  Indices=[2 4 6 8 10 12]  OutputSizes=1
  Subsystem : Subsystem
  Phasors_abc : Outport
  Phasors_Freq : Outport  Port=2
  Phasors_DTFreq : Outport  Port=3
  wires:
  Subsystem/2(Phasors_freq) -> Phasors_Freq/1
  Subsystem/3(Phasors_dtfreq1) -> Phasors_DTFreq/1
  Selector5/1 -> Mux1/1
  Mux1/1 -> Phasors_abc/1
  Selector7/1 -> Mux1/2
  Subsystem/1(Phasors_60Hz) -> Selector5/1, Selector6/1, Selector9/1
  Selector8/1 -> Mux1/4
  Selector6/1 -> Mux1/3
  Measurements/1 -> Subsystem/1(Measurements1)
  Selector9/1 -> Degree to radian1/1(Degree)
  Degree to radian1/1(Radian) -> Selector7/1, Selector8/1

== system Feeder_1/SS_PMU/Subsystem22/Subsystem/Subsystem1 ==
  Measurements : Inport
  Degree to radian1 : Subsystem
  Mux1 : Mux
  Selector5 : Selector  InputPortWidth=12  IndexOptions=Index vector (dialog)  Indices=[1 3 5]  OutputSizes=1
  Selector6 : Selector  InputPortWidth=12  IndexOptions=Index vector (dialog)  Indices=[7 9 11]  OutputSizes=1
  Selector7 : Selector  InputPortWidth=6  IndexOptions=Index vector (dialog)  Indices=[1 2 3]  OutputSizes=1
  Selector8 : Selector  InputPortWidth=6  IndexOptions=Index vector (dialog)  Indices=[4 5 6]  OutputSizes=1
  Selector9 : Selector  InputPortWidth=12  IndexOptions=Index vector (dialog)  Indices=[2 4 6 8 10 12]  OutputSizes=1
  Subsystem : Subsystem
  Phasors_abc : Outport
  Phasors_Freq : Outport  Port=2
  Phasors_DTFreq : Outport  Port=3
  wires:
  Subsystem/2(Phasors_freq) -> Phasors_Freq/1
  Subsystem/3(Phasors_dtfreq1) -> Phasors_DTFreq/1
  Selector5/1 -> Mux1/1
  Mux1/1 -> Phasors_abc/1
  Selector7/1 -> Mux1/2
  Subsystem/1(Phasors_60Hz) -> Selector5/1, Selector6/1, Selector9/1
  Selector8/1 -> Mux1/4
  Selector6/1 -> Mux1/3
  Measurements/1 -> Subsystem/1(Measurements1)
  Selector9/1 -> Degree to radian1/1(Degree)
  Degree to radian1/1(Radian) -> Selector7/1, Selector8/1

== system Feeder_1/SS_PMU/Subsystem3/Subsystem/Subsystem1 ==
  Measurements : Inport
  Degree to radian1 : Subsystem
  Mux1 : Mux
  Selector5 : Selector  InputPortWidth=12  IndexOptions=Index vector (dialog)  Indices=[1 3 5]  OutputSizes=1
  Selector6 : Selector  InputPortWidth=12  IndexOptions=Index vector (dialog)  Indices=[7 9 11]  OutputSizes=1
  Selector7 : Selector  InputPortWidth=6  IndexOptions=Index vector (dialog)  Indices=[1 2 3]  OutputSizes=1
  Selector8 : Selector  InputPortWidth=6  IndexOptions=Index vector (dialog)  Indices=[4 5 6]  OutputSizes=1
  Selector9 : Selector  InputPortWidth=12  IndexOptions=Index vector (dialog)  Indices=[2 4 6 8 10 12]  OutputSizes=1
  Subsystem : Subsystem
  Phasors_abc : Outport
  Phasors_Freq : Outport  Port=2
  Phasors_DTFreq : Outport  Port=3
  wires:
  Subsystem/2(Phasors_freq) -> Phasors_Freq/1
  Subsystem/3(Phasors_dtfreq1) -> Phasors_DTFreq/1
  Selector5/1 -> Mux1/1
  Mux1/1 -> Phasors_abc/1
  Selector7/1 -> Mux1/2
  Subsystem/1(Phasors_60Hz) -> Selector5/1, Selector6/1, Selector9/1
  Selector8/1 -> Mux1/4
  Selector6/1 -> Mux1/3
  Measurements/1 -> Subsystem/1(Measurements1)
  Selector9/1 -> Degree to radian1/1(Degree)
  Degree to radian1/1(Radian) -> Selector7/1, Selector8/1

== system Feeder_1/SS_PMU/Subsystem4/Subsystem/Subsystem1 ==
  Measurements : Inport
  Degree to radian1 : Subsystem
  Mux1 : Mux
  Selector5 : Selector  InputPortWidth=12  IndexOptions=Index vector (dialog)  Indices=[1 3 5]  OutputSizes=1
  Selector6 : Selector  InputPortWidth=12  IndexOptions=Index vector (dialog)  Indices=[7 9 11]  OutputSizes=1
  Selector7 : Selector  InputPortWidth=6  IndexOptions=Index vector (dialog)  Indices=[1 2 3]  OutputSizes=1
  Selector8 : Selector  InputPortWidth=6  IndexOptions=Index vector (dialog)  Indices=[4 5 6]  OutputSizes=1
  Selector9 : Selector  InputPortWidth=12  IndexOptions=Index vector (dialog)  Indices=[2 4 6 8 10 12]  OutputSizes=1
  Subsystem : Subsystem
  Phasors_abc : Outport
  Phasors_Freq : Outport  Port=2
  Phasors_DTFreq : Outport  Port=3
  wires:
  Subsystem/2(Phasors_freq) -> Phasors_Freq/1
  Subsystem/3(Phasors_dtfreq1) -> Phasors_DTFreq/1
  Selector5/1 -> Mux1/1
  Mux1/1 -> Phasors_abc/1
  Selector7/1 -> Mux1/2
  Subsystem/1(Phasors_60Hz) -> Selector5/1, Selector6/1, Selector9/1
  Selector8/1 -> Mux1/4
  Selector6/1 -> Mux1/3
  Measurements/1 -> Subsystem/1(Measurements1)
  Selector9/1 -> Degree to radian1/1(Degree)
  Degree to radian1/1(Radian) -> Selector7/1, Selector8/1

== system Feeder_1/SS_PMU/Subsystem5/Subsystem/Subsystem1 ==
  Measurements : Inport
  Degree to radian1 : Subsystem
  Mux1 : Mux
  Selector5 : Selector  InputPortWidth=12  IndexOptions=Index vector (dialog)  Indices=[1 3 5]  OutputSizes=1
  Selector6 : Selector  InputPortWidth=12  IndexOptions=Index vector (dialog)  Indices=[7 9 11]  OutputSizes=1
  Selector7 : Selector  InputPortWidth=6  IndexOptions=Index vector (dialog)  Indices=[1 2 3]  OutputSizes=1
  Selector8 : Selector  InputPortWidth=6  IndexOptions=Index vector (dialog)  Indices=[4 5 6]  OutputSizes=1
  Selector9 : Selector  InputPortWidth=12  IndexOptions=Index vector (dialog)  Indices=[2 4 6 8 10 12]  OutputSizes=1
  Subsystem : Subsystem
  Phasors_abc : Outport
  Phasors_Freq : Outport  Port=2
  Phasors_DTFreq : Outport  Port=3
  wires:
  Subsystem/2(Phasors_freq) -> Phasors_Freq/1
  Subsystem/3(Phasors_dtfreq1) -> Phasors_DTFreq/1
  Selector5/1 -> Mux1/1
  Mux1/1 -> Phasors_abc/1
  Selector7/1 -> Mux1/2
  Subsystem/1(Phasors_60Hz) -> Selector5/1, Selector6/1, Selector9/1
  Selector8/1 -> Mux1/4
  Selector6/1 -> Mux1/3
  Measurements/1 -> Subsystem/1(Measurements1)
  Selector9/1 -> Degree to radian1/1(Degree)
  Degree to radian1/1(Radian) -> Selector7/1, Selector8/1

== system Feeder_1/SS_PMU/Subsystem6/Subsystem/Subsystem1 ==
  Measurements : Inport
  Degree to radian1 : Subsystem
  Mux1 : Mux
  Selector5 : Selector  InputPortWidth=12  IndexOptions=Index vector (dialog)  Indices=[1 3 5]  OutputSizes=1
  Selector6 : Selector  InputPortWidth=12  IndexOptions=Index vector (dialog)  Indices=[7 9 11]  OutputSizes=1
  Selector7 : Selector  InputPortWidth=6  IndexOptions=Index vector (dialog)  Indices=[1 2 3]  OutputSizes=1
  Selector8 : Selector  InputPortWidth=6  IndexOptions=Index vector (dialog)  Indices=[4 5 6]  OutputSizes=1
  Selector9 : Selector  InputPortWidth=12  IndexOptions=Index vector (dialog)  Indices=[2 4 6 8 10 12]  OutputSizes=1
  Subsystem : Subsystem
  Phasors_abc : Outport
  Phasors_Freq : Outport  Port=2
  Phasors_DTFreq : Outport  Port=3
  wires:
  Subsystem/2(Phasors_freq) -> Phasors_Freq/1
  Subsystem/3(Phasors_dtfreq1) -> Phasors_DTFreq/1
  Selector5/1 -> Mux1/1
  Mux1/1 -> Phasors_abc/1
  Selector7/1 -> Mux1/2
  Subsystem/1(Phasors_60Hz) -> Selector5/1, Selector6/1, Selector9/1
  Selector8/1 -> Mux1/4
  Selector6/1 -> Mux1/3
  Measurements/1 -> Subsystem/1(Measurements1)
  Selector9/1 -> Degree to radian1/1(Degree)
  Degree to radian1/1(Radian) -> Selector7/1, Selector8/1

== system Feeder_1/SS_PMU/Subsystem7/Subsystem/Subsystem1 ==
  Measurements : Inport
  Degree to radian1 : Subsystem
  Mux1 : Mux
  Selector5 : Selector  InputPortWidth=12  IndexOptions=Index vector (dialog)  Indices=[1 3 5]  OutputSizes=1
  Selector6 : Selector  InputPortWidth=12  IndexOptions=Index vector (dialog)  Indices=[7 9 11]  OutputSizes=1
  Selector7 : Selector  InputPortWidth=6  IndexOptions=Index vector (dialog)  Indices=[1 2 3]  OutputSizes=1
  Selector8 : Selector  InputPortWidth=6  IndexOptions=Index vector (dialog)  Indices=[4 5 6]  OutputSizes=1
  Selector9 : Selector  InputPortWidth=12  IndexOptions=Index vector (dialog)  Indices=[2 4 6 8 10 12]  OutputSizes=1
  Subsystem : Subsystem
  Phasors_abc : Outport
  Phasors_Freq : Outport  Port=2
  Phasors_DTFreq : Outport  Port=3
  wires:
  Subsystem/2(Phasors_freq) -> Phasors_Freq/1
  Subsystem/3(Phasors_dtfreq1) -> Phasors_DTFreq/1
  Selector5/1 -> Mux1/1
  Mux1/1 -> Phasors_abc/1
  Selector7/1 -> Mux1/2
  Subsystem/1(Phasors_60Hz) -> Selector5/1, Selector6/1, Selector9/1
  Selector8/1 -> Mux1/4
  Selector6/1 -> Mux1/3
  Measurements/1 -> Subsystem/1(Measurements1)
  Selector9/1 -> Degree to radian1/1(Degree)
  Degree to radian1/1(Radian) -> Selector7/1, Selector8/1

== system Feeder_1/SS_PMU/Subsystem8/Subsystem/Subsystem1 ==
  Measurements : Inport
  Degree to radian1 : Subsystem
  Mux1 : Mux
  Selector5 : Selector  InputPortWidth=12  IndexOptions=Index vector (dialog)  Indices=[1 3 5]  OutputSizes=1
  Selector6 : Selector  InputPortWidth=12  IndexOptions=Index vector (dialog)  Indices=[7 9 11]  OutputSizes=1
  Selector7 : Selector  InputPortWidth=6  IndexOptions=Index vector (dialog)  Indices=[1 2 3]  OutputSizes=1
  Selector8 : Selector  InputPortWidth=6  IndexOptions=Index vector (dialog)  Indices=[4 5 6]  OutputSizes=1
  Selector9 : Selector  InputPortWidth=12  IndexOptions=Index vector (dialog)  Indices=[2 4 6 8 10 12]  OutputSizes=1
  Subsystem : Subsystem
  Phasors_abc : Outport
  Phasors_Freq : Outport  Port=2
  Phasors_DTFreq : Outport  Port=3
  wires:
  Subsystem/2(Phasors_freq) -> Phasors_Freq/1
  Subsystem/3(Phasors_dtfreq1) -> Phasors_DTFreq/1
  Selector5/1 -> Mux1/1
  Mux1/1 -> Phasors_abc/1
  Selector7/1 -> Mux1/2
  Subsystem/1(Phasors_60Hz) -> Selector5/1, Selector6/1, Selector9/1
  Selector8/1 -> Mux1/4
  Selector6/1 -> Mux1/3
  Measurements/1 -> Subsystem/1(Measurements1)
  Selector9/1 -> Degree to radian1/1(Degree)
  Degree to radian1/1(Radian) -> Selector7/1, Selector8/1

== system Feeder_1/SS_PMU/Subsystem9/Subsystem/Subsystem1 ==
  Measurements : Inport
  Degree to radian1 : Subsystem
  Mux1 : Mux
  Selector5 : Selector  InputPortWidth=12  IndexOptions=Index vector (dialog)  Indices=[1 3 5]  OutputSizes=1
  Selector6 : Selector  InputPortWidth=12  IndexOptions=Index vector (dialog)  Indices=[7 9 11]  OutputSizes=1
  Selector7 : Selector  InputPortWidth=6  IndexOptions=Index vector (dialog)  Indices=[1 2 3]  OutputSizes=1
  Selector8 : Selector  InputPortWidth=6  IndexOptions=Index vector (dialog)  Indices=[4 5 6]  OutputSizes=1
  Selector9 : Selector  InputPortWidth=12  IndexOptions=Index vector (dialog)  Indices=[2 4 6 8 10 12]  OutputSizes=1
  Subsystem : Subsystem
  Phasors_abc : Outport
  Phasors_Freq : Outport  Port=2
  Phasors_DTFreq : Outport  Port=3
  wires:
  Subsystem/2(Phasors_freq) -> Phasors_Freq/1
  Subsystem/3(Phasors_dtfreq1) -> Phasors_DTFreq/1
  Selector5/1 -> Mux1/1
  Mux1/1 -> Phasors_abc/1
  Selector7/1 -> Mux1/2
  Subsystem/1(Phasors_60Hz) -> Selector5/1, Selector6/1, Selector9/1
  Selector8/1 -> Mux1/4
  Selector6/1 -> Mux1/3
  Measurements/1 -> Subsystem/1(Measurements1)
  Selector9/1 -> Degree to radian1/1(Degree)
  Degree to radian1/1(Radian) -> Selector7/1, Selector8/1

== system Feeder_1/SM_NG/Dynamic Load BCDC2/Single-Phase Dynamic Load1/model/Break  Alg. Loop1 ==
  In : Inport
  Complex to Real-Imag : ComplexToRealImag
  Real-Imag to Complex : RealImagToComplex
  imag : simulink_extras/Additional Linear/Transfer Fcn (with initial outputs)  N=[1]  D="[100e-6  1]"  Y0=imag(I1_init*exp(-j*Pha_V0*pi/180))  U0=imag(I1_init*exp(-j*Pha_V0*pi/180))
  real : simulink_extras/Additional Linear/Transfer Fcn (with initial outputs)  N=[1]  D="[100e-6  1]"  Y0=real(I1_init*exp(-j*Pha_V0*pi/180))  U0=real(I1_init*exp(-j*Pha_V0*pi/180))
  Out : Outport
  wires:
  Complex to Real-Imag/2 -> imag/1
  Complex to Real-Imag/1 -> real/1
  Real-Imag to Complex/1 -> Out/1
  In/1 -> Complex to Real-Imag/1
  imag/1 -> Real-Imag to Complex/2
  real/1 -> Real-Imag to Complex/1
